simulink model "Robust_controller_2"  (R2020b)
settings: Solver=VariableStepAuto  StartTime=0.0  StopTime=50  RelTol=1e-3
InitFcn:
  | % reference input
  | qref_1 = 1;
  | qref_2 = 2;
  | 
  | % generator parameters
  | A_1 = 1;
  | A_2 = 1;
  | psi_1 = 0;
  | psi_2 = 0;
  | omegaref_1 = 1;
  | omegaref_2 = 2;
  | 
  | wref_0 = [A_1*sin(psi_1) omegaref_1*A_1*cos(psi_1) A_2*sin(psi_2) omegaref_2*A_2*cos(psi_2)];
  | Sref = [0 1 0 0; -omegaref_1^2 0 0 0 ; 0 0 0 1; 0 0 -omegaref_2^2 0];
  | Qrefp = [1 0 0 0; 0 0 1 0];
  | Qrefv = [0 1 0 0 ; 0 0 0 1];
  | Qrefa = [-omegaref_1^2 0 0 0; 0 0 -omegaref_2^2 0];
  | 
  | % model parameters
  | m_1 = 1;
  | m_2 = 1;
  | l_1 = 1;
  | l_2 = 1;
  | l_c1 = 1/2;
  | l_c2 = 1/2;
  | I_1 = 1;
  | I_2 = 1;
  | g = 9.81;
  | 
  | rho_1 = m_1*l_c1^2+m_2*l_1^2+2*m_2*l_1*l_c2^2+I_1;
  | rho_2 = m_2*l_c2^2+I_2;
  | rho_3 = m_2*l_1*l_c2;
  | rho_4 = (m_1*l_c1+m_2*l_1)*g;
  | rho_5 = m_2*l_c2*g;
  | rho_6 = m_2*l_c2;
  | 
  | % friction
  | F_fric = [0.1 0; 0 0.1];
  | 
  | % observer parameters
  | H_p = [10 1; 1 10];
  | H_v = [30 3; 3 30];
  | H_s =  [30 3; 3 30];
  | 
  | % check eigen values
  | P = [-H_p eye(2) zeros(2); -H_v zeros(2) eye(2); -H_s zeros(2) zeros(2)];
  | eig(P)
  | 
  | % control law coefficients
  | kappa = 1000;
  | K = [1 0 1 0; 0 1 0 1];
  | N = inf;
  | M_0 = [rho_1+rho_2+2*rho_3*cos(qref_2) rho_2+rho_3*cos(qref_2); rho_2+rho_3*cos(qref_2) rho_2];
  | 
  | % disturbance generator parameters
  | omega_dist_1 = 1;
  | omega_dist_2 = 2;
  | amp_dist_1 = 30;
  | amp_dist_2 = 40;
  | bias_dist_1 = 5;
  | bias_dist_2 = 6;
  | phase_dist_1 = 7;
  | phase_dist_2 = 8;
  | 
  | S_dist_1 = [0 0 0; 0 0 1; 0 -omega_dist_1^2 0];
  | S_dist_2 = [0 0 0; 0 0 1; 0 -omega_dist_2^2 0];
  | 
  | S_dist = blkdiag(S_dist_1, S_dist_2);
  | w_dist_0 = [bias_dist_1; amp_dist_1*sin(phase_dist_1); omega_dist_1*amp_dist_1*cos(phase_dist_1);
  | bias_dist_2; amp_dist_2*sin(phase_dist_2); omega_dist_2*amp_dist_2*cos(phase_dist_2)];
  | H_dist_1 = [1 1 0];
  | H_dist_2 = [1 1 0];
  | H_dist = blkdiag(H_dist_1, H_dist_2);
  | 
  | % internal model parameters
  | F_1 = [zeros(2, 1) eye(2); -1 -3 -3];
  | F_2 = [zeros(2, 1) eye(2); -1 -3 -3];
  | 
  | G_1 = [zeros(2, 1); 1];
  | G_2 = [zeros(2, 1); 1];
  | 
  | F = blkdiag(F_1, F_2);
  | G = blkdiag(G_1, G_2);
  | 
  | Gamma_1 = -F_1(3, :)-[0 omega_dist_1^2 0];
  | Gamma_2 = -F_2(3, :)-[0 omega_dist_2^2 0];
  | Gamma = blkdiag(Gamma_1, Gamma_2);
settings Model: Creator=Eugene  LastModifiedBy=Eugene

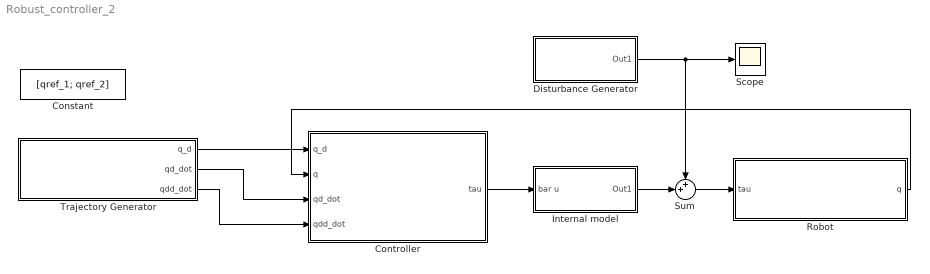
== system Robust_controller_2 ==
  Constant : Constant  Value=[qref_1; qref_2]
  Controller : Subsystem
  Disturbance Generator : Subsystem
  Internal model : Subsystem
  Robot : Subsystem
  Scope : Scope
  Sum : Sum  Inputs=++|
  Trajectory Generator : Subsystem
  wires:
  Robot/1(q) -> Controller/2(q)
  Controller/1(tau) -> Internal model/1(bar u)
  Internal model/1(Out1) -> Sum/2
  Sum/1 -> Robot/1(tau)
  Disturbance Generator/1(Out1) -> Sum/1, Scope/1
  Trajectory Generator/1(q_d) -> Controller/1(q_d)
  Trajectory Generator/2(qd_dot) -> Controller/3(qd_dot)
  Trajectory Generator/3(qdd_dot) -> Controller/4(qdd_dot)

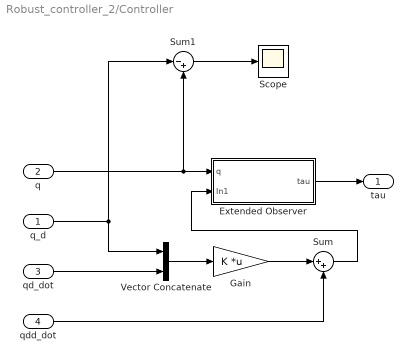
== system Robust_controller_2/Controller ==
  q_d : Inport
  q : Inport  Port=2
  qd_dot : Inport  Port=3
  qdd_dot : Inport  Port=4
  Extended Observer : Subsystem
  Gain : Gain  Gain=K  Multiplication=Matrix(K*u) (u vector)
  Scope : Scope
  Sum : Sum  Inputs=|++
  Sum1 : Sum  Inputs=|-+
  Vector Concatenate : Concatenate  ConcatenateDimension=2
  tau : Outport
  wires:
  Sum1/1 -> Scope/1
  q/1 -> Extended Observer/1(q), Sum1/2
  qd_dot/1 -> Vector Concatenate/2
  Vector Concatenate/1 -> Gain/1
  Gain/1 -> Sum/1
  qdd_dot/1 -> Sum/2
  Extended Observer/1(tau) -> tau/1
  Sum/1 -> Extended Observer/2(In1)
  q_d/1 -> Sum1/1, Vector Concatenate/1

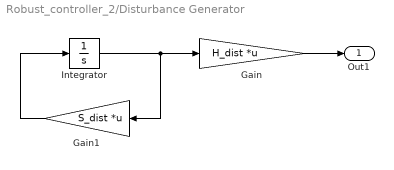
== system Robust_controller_2/Disturbance Generator ==
  Gain : Gain  Gain=H_dist  Multiplication=Matrix(K*u) (u vector)
  Gain1 : Gain  Gain=S_dist  Multiplication=Matrix(K*u) (u vector)
  Integrator : Integrator  InitialCondition=w_dist_0
  Out1 : Outport
  wires:
  Gain/1 -> Out1/1
  Integrator/1 -> Gain1/1, Gain/1
  Gain1/1 -> Integrator/1

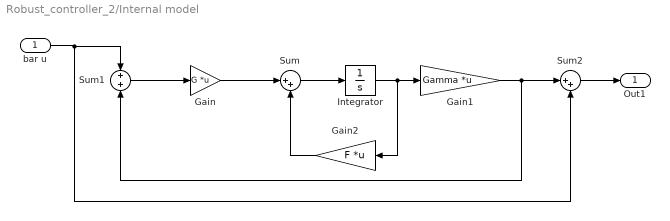
== system Robust_controller_2/Internal model ==
  bar u : Inport
  Gain : Gain  Gain=G  Multiplication=Matrix(K*u)
  Gain1 : Gain  Gain=Gamma  Multiplication=Matrix(K*u)
  Gain2 : Gain  Gain=F  Multiplication=Matrix(K*u) (u vector)
  Integrator : Integrator
  Sum : Sum  Inputs=|++
  Sum1 : Sum
  Sum2 : Sum  Inputs=|++
  Out1 : Outport
  wires:
  bar u/1 -> Sum2/2, Sum1/1
  Sum1/1 -> Gain/1
  Gain/1 -> Sum/1
  Sum/1 -> Integrator/1
  Sum2/1 -> Out1/1
  Integrator/1 -> Gain2/1, Gain1/1
  Gain1/1 -> Sum1/2, Sum2/1
  Gain2/1 -> Sum/2

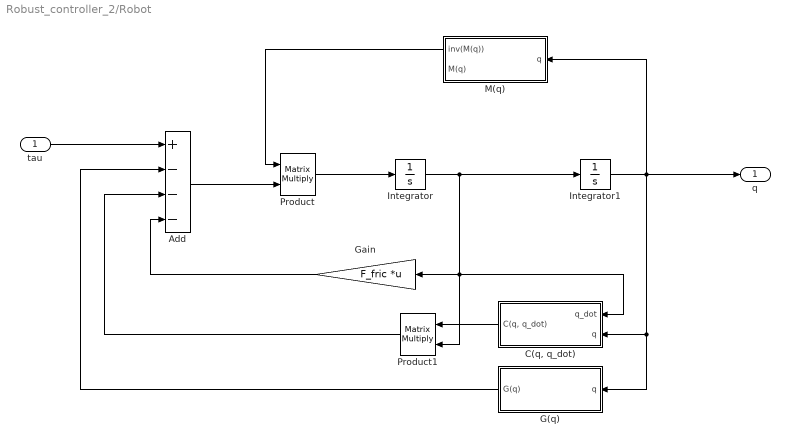
== system Robust_controller_2/Robot ==
  tau : Inport
  Add : Sum  Inputs=+---
  "C(q, q_dot)" : Subsystem
  G(q) : Subsystem
  Gain : Gain  Gain=F_fric  Multiplication=Matrix(K*u) (u vector)
  Integrator : Integrator
  Integrator1 : Integrator
  M(q) : Subsystem
  Product : Product  Multiplication=Matrix(*)
  Product1 : Product  Multiplication=Matrix(*)
  q : Outport
  wires:
  Integrator1/1 -> q/1, "C(q, q_dot)"/2(q), G(q)/1(q), M(q)/1(q)
  Integrator/1 -> "C(q, q_dot)"/1(q_dot), Product1/2, Gain/1, Integrator1/1
  M(q)/1(inv(M(q))) -> Product/1
  Product1/1 -> Add/3
  tau/1 -> Add/1
  "C(q, q_dot)"/1("C(q, q_dot)") -> Product1/1
  Add/1 -> Product/2
  G(q)/1(G(q)) -> Add/2
  Product/1 -> Integrator/1
  Gain/1 -> Add/4

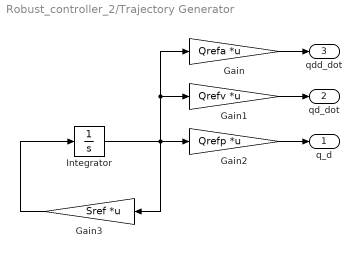
== system Robust_controller_2/Trajectory Generator ==
  Gain : Gain  Gain=Qrefa  Multiplication=Matrix(K*u) (u vector)
  Gain1 : Gain  Gain=Qrefv  Multiplication=Matrix(K*u) (u vector)
  Gain2 : Gain  Gain=Qrefp  Multiplication=Matrix(K*u) (u vector)
  Gain3 : Gain  Gain=Sref  Multiplication=Matrix(K*u) (u vector)
  Integrator : Integrator  InitialCondition=wref_0
  q_d : Outport
  qd_dot : Outport  Port=2
  qdd_dot : Outport  Port=3
  wires:
  Gain3/1 -> Integrator/1
  Integrator/1 -> Gain3/1, Gain1/1, Gain/1, Gain2/1
  Gain2/1 -> q_d/1
  Gain1/1 -> qd_dot/1
  Gain/1 -> qdd_dot/1

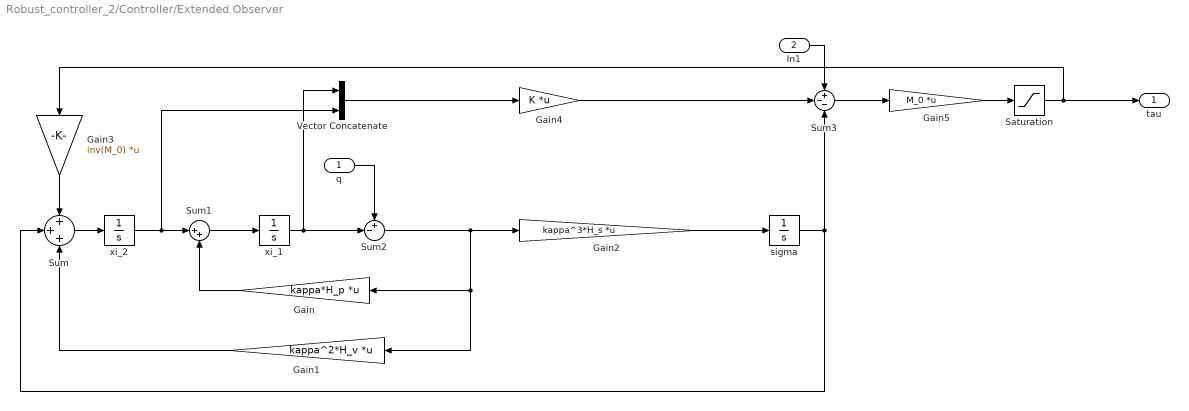
== system Robust_controller_2/Controller/Extended Observer ==
  q : Inport
  In1 : Inport  Port=2
  Gain : Gain  Gain=kappa*H_p  Multiplication=Matrix(K*u) (u vector)
  Gain1 : Gain  Gain=kappa^2*H_v  Multiplication=Matrix(K*u) (u vector)
  Gain2 : Gain  Gain=kappa^3*H_s  Multiplication=Matrix(K*u) (u vector)
  Gain3 : Gain  Gain=inv(M_0)  Multiplication=Matrix(K*u) (u vector)
  Gain4 : Gain  Gain=K  Multiplication=Matrix(K*u) (u vector)
  Gain5 : Gain  Gain=M_0  Multiplication=Matrix(K*u) (u vector)
  Saturation : Saturate  UpperLimit=N  LowerLimit=-N
  Sum : Sum  Inputs=+++
  Sum1 : Sum  Inputs=|++
  Sum2 : Sum  Inputs=+-|
  Sum3 : Sum  Inputs=+--
  Vector Concatenate : Concatenate  ConcatenateDimension=2
  sigma : Integrator
  xi_1 : Integrator
  xi_2 : Integrator
  tau : Outport
  wires:
  Sum/1 -> xi_2/1
  xi_2/1 -> Vector Concatenate/2, Sum1/1
  Sum1/1 -> xi_1/1
  Gain/1 -> Sum1/2
  Gain2/1 -> sigma/1
  xi_1/1 -> Vector Concatenate/1, Sum2/2
  q/1 -> Sum2/1
  Sum2/1 -> Gain/1, Gain1/1, Gain2/1
  Gain1/1 -> Sum/3
  Gain3/1 -> Sum/1
  Vector Concatenate/1 -> Gain4/1
  Gain4/1 -> Sum3/2
  In1/1 -> Sum3/1
  sigma/1 -> Sum/2, Sum3/3
  Sum3/1 -> Gain5/1
  Gain5/1 -> Saturation/1
  Saturation/1 -> Gain3/1, tau/1

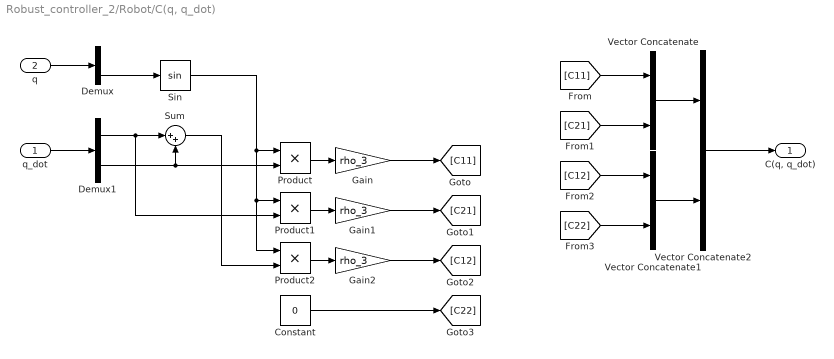
== system Robust_controller_2/Robot/C(q, q_dot) ==
  q_dot : Inport
  q : Inport  Port=2
  Constant : Constant  Value=0
  Demux : Demux  Outputs=2
  Demux1 : Demux  Outputs=2
  Gain : Gain  Gain=rho_3
  Gain1 : Gain  Gain=rho_3
  Gain2 : Gain  Gain=rho_3
  Product : Product
  Product1 : Product
  Product2 : Product
  Sin : Trigonometry
  Sum : Sum  Inputs=|++
  Vector Concatenate : Concatenate
  Vector Concatenate1 : Concatenate
  Vector Concatenate2 : Concatenate  Mode=Multidimensional array  ConcatenateDimension=2
  "C(q, q_dot)" : Outport
  wires:
  q/1 -> Demux/1
  q_dot/1 -> Demux1/1
  Demux1/1 -> Sum/1, Product1/2
  Sin/1 -> Product/1, Product2/1, Product1/1
  Demux1/2 -> Product/2, Sum/2
  Sum/1 -> Product2/2
  Product/1 -> Gain/1
  Product1/1 -> Gain1/1
  Product2/1 -> Gain2/1
  Gain/1 -> [C11]
  Gain1/1 -> [C21]
  Gain2/1 -> [C12]
  Constant/1 -> [C22]
  [C12] -> Vector Concatenate1/1
  [C22] -> Vector Concatenate1/2
  [C21] -> Vector Concatenate/2
  [C11] -> Vector Concatenate/1
  Vector Concatenate2/1 -> "C(q, q_dot)"/1
  Vector Concatenate/1 -> Vector Concatenate2/1
  Vector Concatenate1/1 -> Vector Concatenate2/2
  Demux/2 -> Sin/1

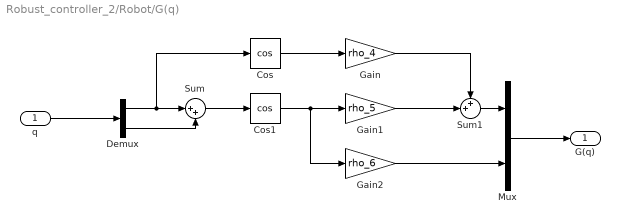
== system Robust_controller_2/Robot/G(q) ==
  q : Inport
  Cos : Trigonometry  Operator=cos
  Cos1 : Trigonometry  Operator=cos
  Demux : Demux  Outputs=2
  Gain : Gain  Gain=rho_4
  Gain1 : Gain  Gain=rho_5
  Gain2 : Gain  Gain=rho_6
  Mux : Mux  Inputs=2
  Sum : Sum  Inputs=|++
  Sum1 : Sum  Inputs=++|
  G(q) : Outport
  wires:
  q/1 -> Demux/1
  Demux/1 -> Cos/1, Sum/1
  Demux/2 -> Sum/2
  Sum/1 -> Cos1/1
  Cos/1 -> Gain/1
  Cos1/1 -> Gain2/1, Gain1/1
  Gain/1 -> Sum1/1
  Gain1/1 -> Sum1/2
  Sum1/1 -> Mux/1
  Gain2/1 -> Mux/2
  Mux/1 -> G(q)/1

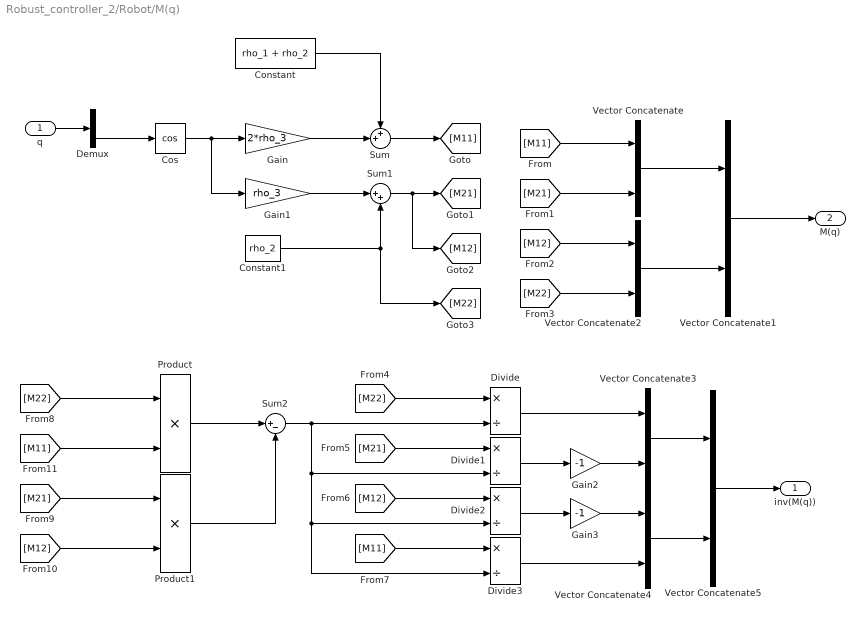
== system Robust_controller_2/Robot/M(q) ==
  q : Inport
  Constant : Constant  Value=rho_1 + rho_2
  Constant1 : Constant  Value=rho_2
  Cos : Trigonometry  Operator=cos
  Demux : Demux  Outputs=2
  Divide{,1..3} (4 alike) : Product  Inputs=*/
  Gain : Gain  Gain=2*rho_3
  Gain1 : Gain  Gain=rho_3
  Gain2 : Gain  Gain=-1
  Gain3 : Gain  Gain=-1
  Product : Product
  Product1 : Product
  Sum : Sum  Inputs=++|
  Sum1 : Sum  Inputs=|++
  Sum2 : Sum  Inputs=|+-
  Vector Concatenate : Concatenate
  Vector Concatenate1 : Concatenate  Mode=Multidimensional array  ConcatenateDimension=2
  Vector Concatenate2 : Concatenate
  Vector Concatenate3 : Concatenate  Mode=Multidimensional array  ConcatenateDimension=2
  Vector Concatenate4 : Concatenate  Mode=Multidimensional array  ConcatenateDimension=2
  Vector Concatenate5 : Concatenate  Mode=Multidimensional array
  inv(M(q)) : Outport
  M(q) : Outport  Port=2
  wires:
  q/1 -> Demux/1
  Cos/1 -> Gain1/1, Gain/1
  Gain/1 -> Sum/2
  Constant/1 -> Sum/1
  Sum1/1 -> [M12], [M21]
  Sum/1 -> [M11]
  Gain1/1 -> Sum1/1
  Constant1/1 -> [M22], Sum1/2
  [M21] -> Product1/1
  [M11] -> Product/2
  [M12] -> Product1/2
  [M22] -> Product/1
  Product/1 -> Sum2/1
  Product1/1 -> Sum2/2
  [M21] -> Divide1/1
  [M22] -> Divide/1
  [M11] -> Divide3/1
  [M12] -> Divide2/1
  Sum2/1 -> Divide1/2, Divide2/2, Divide3/2, Divide/2
  Divide1/1 -> Gain2/1
  Divide2/1 -> Gain3/1
  Divide/1 -> Vector Concatenate3/1
  Gain2/1 -> Vector Concatenate3/2
  Divide3/1 -> Vector Concatenate4/2
  Gain3/1 -> Vector Concatenate4/1
  Vector Concatenate3/1 -> Vector Concatenate5/1
  Vector Concatenate4/1 -> Vector Concatenate5/2
  Vector Concatenate5/1 -> inv(M(q))/1
  [M11] -> Vector Concatenate/1
  [M22] -> Vector Concatenate2/2
  [M12] -> Vector Concatenate2/1
  [M21] -> Vector Concatenate/2
  Vector Concatenate/1 -> Vector Concatenate1/1
  Vector Concatenate2/1 -> Vector Concatenate1/2
  Vector Concatenate1/1 -> M(q)/1
  Demux/2 -> Cos/1
